simulink model "w1p1"  (R2020a)
settings: Solver=VariableStepAuto  StartTime=0.0  StopTime=10  RelTol=1e-3
values from neighbouring files (symbols this model uses):
  B = 50    [p1.mat]    (also in w1p1.mat)
  K1 = 50    [p1.mat]    (also in w1p1.mat)
  K12 = 25    [w1p1.mat]
  M1 = 100    [p1.mat]    (also in w1p1.mat)
  M2 = 5    [w1p1.mat]
settings Model: Creator=Shubham  LastModifiedBy=Shubham

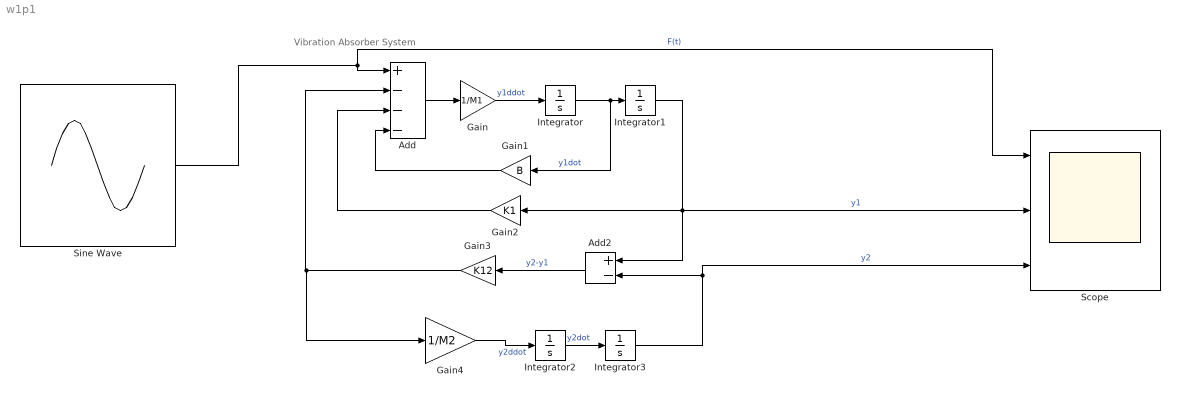
== system w1p1 ==
  note: Vibration Absorber System
  Add : Sum  Inputs=+---
  Add2 : Sum  Inputs=+-
  Gain : Gain  Gain=1/M1
  Gain1 : Gain  Gain=B
  Gain2 : Gain  Gain=K1
  Gain3 : Gain  Gain=K12
  Gain4 : Gain  Gain=1/M2
  Integrator : Integrator  InitialCondition=1
  Integrator1 : Integrator
  Integrator2 : Integrator
  Integrator3 : Integrator
  Scope : Scope  NumInputPorts=3
  Sine Wave : Sin  Amplitude=2  Frequency=10*2*pi  SampleTime=5e-3
  wires:
  Gain1/1 -> Add/4
  Gain2/1 -> Add/3
  Gain3/1 -> Gain4/1, Add/2
  Add2/1 -> Gain3/1  "y2-y1"
  Sine Wave/1 -> Scope/1, Add/1  "F(t)"
  Add/1 -> Gain/1
  Gain/1 -> Integrator/1  "y1ddot"
  Integrator2/1 -> Integrator3/1  "y2dot"
  Integrator1/1 -> Add2/1, Scope/2, Gain2/1  "y1"
  Gain4/1 -> Integrator2/1  "y2ddot"
  Integrator3/1 -> Add2/2, Scope/3  "y2"
  Integrator/1 -> Integrator1/1, Gain1/1  "y1dot"
